simulink subsystem "RT_SkewCalculation_V1_2"  (R2025a)
settings: Solver=VariableStepAuto  StartTime=0.0  StopTime=2  RelTol=1e-3
model mask{RT_RotorRadius=0}
  mask prompts: RT_RotorRadius "Rotor radius [m]"
libraries: aerolibutil x1
settings Model: DefaultTestHarness=RT_SkewCalculation_V1_0_Harness2  Creator=Admin  LastModifiedBy=Admin
settings DataIOCC: OutputSaveName=simout

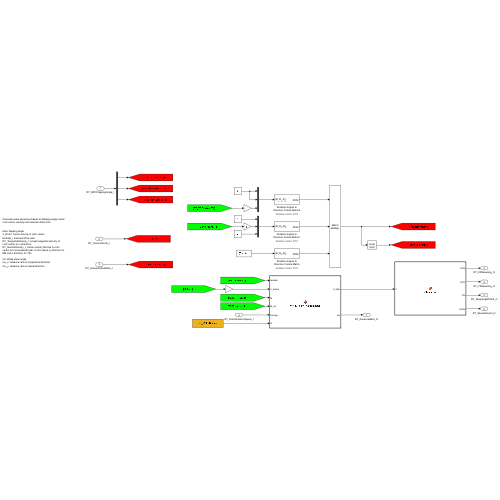
[thumbnail: Simulink's stored preview of the top-level diagram]
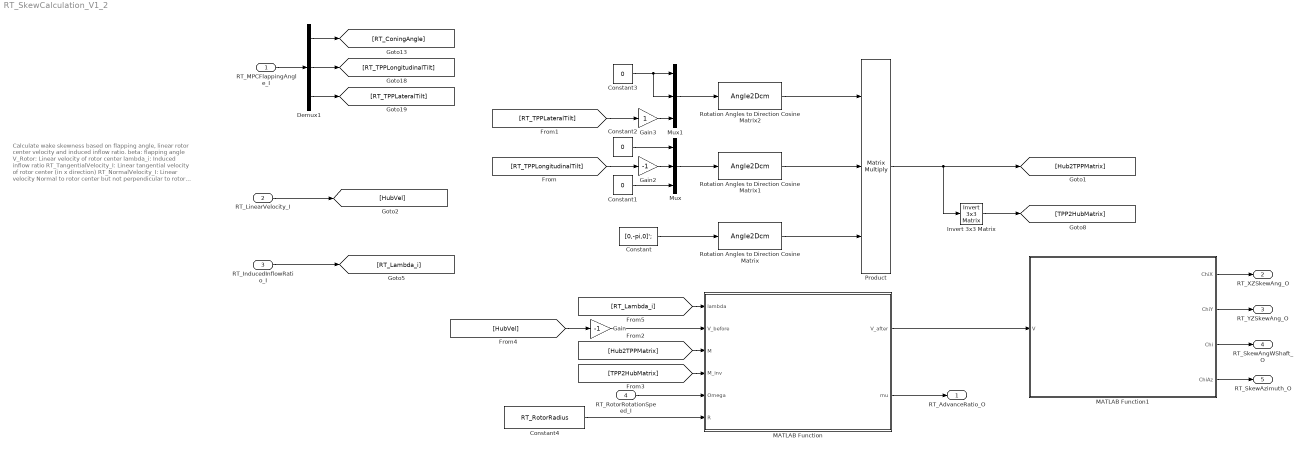
== system RT_SkewCalculation_V1_2 ==
  note: Calculate wake skewness based on flapping angle, linear rotor center velocity and induced inflow ratio.
      |
      | beta: flapping angle
      | V_Rotor: Linear velocity of rotor center
      | lambda_i: Induced inflow ratio
      | RT_TangentialVelocity_I: Linear tangential velocity of rotor center (in x direction)
      | RT_NormalVelocity_I: Linear velocity Normal to rotor center but not perpendicular to rotor plane (y direction for MR and z direction for TR)
      |
      | chi: Wake skew angle
      | mu_x: advance ratio in longitudinal direction
      | mu_y: advance ratio in lateral direction
  RT_MPCFlappingAngle_I : Inport
  RT_LinearVelocity_I : Inport  Port=2
  RT_InducedInflowRatio_I : Inport  Port=3
  RT_RotorRotationSpeed_I : Inport  Port=4
  Constant : Constant  Value=[0,-pi,0]';
  Constant1 : Constant  Value=0
  Constant2 : Constant  Value=0
  Constant3 : Constant  Value=0
  Constant4 : Constant  Value=RT_RotorRadius
  Demux1 : Demux  Outputs=3
  Gain : Gain  Gain=-1
  Gain2 : Gain  Gain=-1
  Gain3 : Gain
  Invert 3x3 Matrix : aerolibutil/Invert  3x3 Matrix
  MATLAB Function : MATLAB Function  TreatAsAtomicUnit=on
  MATLAB Function1 : MATLAB Function  TreatAsAtomicUnit=on
  Mux : Mux  Inputs=3
  Mux1 : Mux  Inputs=3
  Product : Product  Inputs=3  Multiplication=Matrix(*)
  Rotation Angles to Direction Cosine Matrix : Angle2Dcm
      settings: AttributesFormatString=Rotation Order: %<rotationOrder>
  Rotation Angles to Direction Cosine Matrix1 : Angle2Dcm
      settings: AttributesFormatString=Rotation Order: %<rotationOrder>
  Rotation Angles to Direction Cosine Matrix2 : Angle2Dcm
      settings: AttributesFormatString=Rotation Order: %<rotationOrder>
  RT_AdvanceRatio_O : Outport
  RT_XZSkewAng_O : Outport  Port=2
  RT_YZSkewAng_O : Outport  Port=3
  RT_SkewAngWShaft_O : Outport  Port=4
  RT_SkewAzimuth_O : Outport  Port=5
  wires:
  Constant1/1 -> Mux/3
  [Hub2TPPMatrix] -> MATLAB Function/3(M)
  RT_LinearVelocity_I/1 -> [HubVel]
  [RT_TPPLongitudinalTilt] -> Gain2/1
  Rotation Angles to Direction Cosine Matrix/1 -> Product/3
  Rotation Angles to Direction Cosine Matrix2/1 -> Product/1
  RT_MPCFlappingAngle_I/1 -> Demux1/1
  Constant4/1 -> MATLAB Function/6(R)
  Constant/1 -> Rotation Angles to Direction Cosine Matrix/1
  Mux1/1 -> Rotation Angles to Direction Cosine Matrix2/1
  [TPP2HubMatrix] -> MATLAB Function/4(M_inv)
  MATLAB Function1/2(ChiY) -> RT_YZSkewAng_O/1
  Gain2/1 -> Mux/2
  MATLAB Function1/3(Chi) -> RT_SkewAngWShaft_O/1
  [RT_TPPLateralTilt] -> Gain3/1
  Mux/1 -> Rotation Angles to Direction Cosine Matrix1/1
  Rotation Angles to Direction Cosine Matrix1/1 -> Product/2
  Demux1/2 -> [RT_TPPLongitudinalTilt]
  Constant3/1 -> Mux1/1, Mux1/2
  MATLAB Function/2(mu) -> RT_AdvanceRatio_O/1
  Gain3/1 -> Mux1/3
  MATLAB Function1/4(ChiAz) -> RT_SkewAzimuth_O/1
  [HubVel] -> Gain/1
  Demux1/3 -> [RT_TPPLateralTilt]
  Constant2/1 -> Mux/1
  RT_InducedInflowRatio_I/1 -> [RT_Lambda_i]
  RT_RotorRotationSpeed_I/1 -> MATLAB Function/5(Omega)
  MATLAB Function1/1(ChiX) -> RT_XZSkewAng_O/1
  Invert 3x3 Matrix/1 -> [TPP2HubMatrix]
  MATLAB Function/1(V_after) -> MATLAB Function1/1(V)
  Demux1/1 -> [RT_ConingAngle]
  Product/1 -> Invert 3x3 Matrix/1, [Hub2TPPMatrix]
  [RT_Lambda_i] -> MATLAB Function/1(lambda)
  Gain/1 -> MATLAB Function/2(V_before)

== matlab function RT_SkewCalculation_V1_2/MATLAB Function1 ==
  data: V input; ChiX output; ChiY output; Chi output; ChiAz output
function [ChiX,ChiY,Chi,ChiAz] = Skewness(V)
u = -V(1);
v = V(2);
w = V(3);
ChiAz = atan2(v,u);
if ChiAz < 0
    ChiAz = ChiAz+2*pi;
end
Chi = atan2(sqrt(v^2+u^2),w);
ChiX = atan2(u,w);
ChiY = atan2(v,w);

== matlab function RT_SkewCalculation_V1_2/MATLAB Function ==
  data: lambda input; V_after output; V_before input; M input; M_inv input; Omega input; R input; mu output
function [V_after,mu] = WindVelocityThroughRotor(lambda, V_before, M, M_inv, Omega, R)

V_TPP = M*V_before;
V_after = M_inv*(V_TPP+[0;0;-Omega*R*lambda]);
mu = V_TPP/Omega/R;
